simulink model "celp_ex_lsf"  (Simulink 6.1)
settings: Solver=FixedStepDiscrete  SolverMode=SingleTasking  StartTime=0.0  StopTime=300  RelTol=1e-3
PreLoadFcn:
  | load lpcvocoder.mat;
undefined symbols (not defined in the file): jet, magnitude, poly2lsf
libraries: simulink x16, dspcelplib x12, dspindex x9, dspstat3 x8, dspbuff3 x8, dspquant2 x6, dspmtrx3 x6, dsparch4 x4, dspsigops x4, dspmathops x4, dsplp x3, dspspect3 x3
(part 1 of 2)
settings Model: RequirementInfo=9  CovMetricSettings=d  Creator=The MathWorks Inc.  LastModifiedBy=igor  ExtModeTrigMode=oneshot  ExtModeArmWhenConnect=off  ExtModeAutoUpdateStatusClock=off  ProdHWDeviceType=Specified
settings DataIOCC: LimitDataPoints=off  SaveFormat=Structure  SaveOutput=off  SaveTime=off  SignalLoggingName=sigsOut
settings OptimizationCC: BlockReduction=off  BooleanDataType=off  InlineInvariantSignals=off
settings DebuggingCC: CheckExecutionContextPreStartOutputMsg=on  CheckExecutionContextRuntimeOutputMsg=on  InheritedTsInSrcMsg=none  IntegerOverflowMsg=none
settings HardwareCC: ProdHWDeviceType=Specified

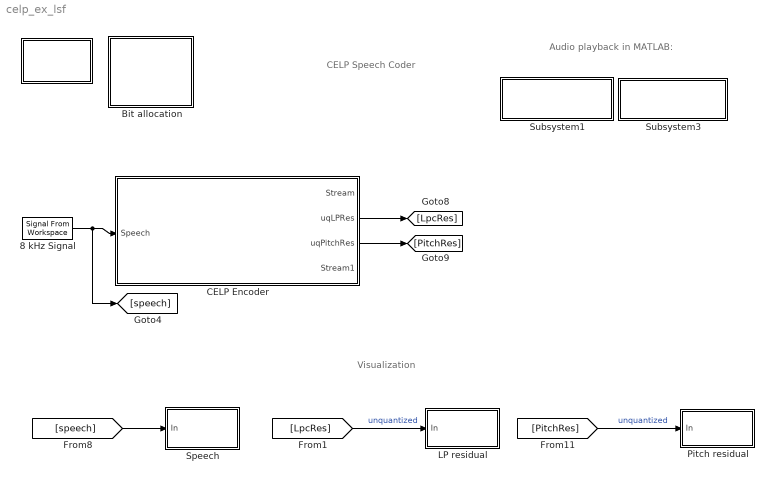
== system celp_ex_lsf ==
  note: CELP Speech Coder
  note: Visualization
  note: Audio playback in MATLAB:
  " " : Subsystem
      mask Type: CELP Coder Demo Info
      mask Display: disp('Info')
  "  Bit allocation" : Subsystem  mask(Bit Allocation){bitLSF1to3=10, bitLSF4to6=10, bitLSF7to10=10, bitD=7, bitBeta=6, bitSignGain=4, bitPhase=17, bitAlpha=6}
      mask prompts: bitLSF1to3 "Number of bits for 1st LSF subvector (1 to 3) (per frame):"; bitLSF4to6 "Number of bits for 2nd LSF subvector (4 to 6) (per frame):"; bitLSF7to10 "Number of bits for 3rd LSF subvector (7 to 10) (per frame):"; bitD "Number of bits for Pitch Delay, D (per subframe):"; bitBeta "Number of bits for Pitch Gain, Beta (per subframe):"; bitSignGain "Number of bits for sign of 4 FCB pulses (per subframe):"; bitPhase "Number of bits for position of 4 FCB pulses (per subframe):"; bitAlpha "Number of bits for FCB Gain, Alpha (per subframe):"
      mask help: Bit allocation for the speech coder designed for narrowband speech (sampling frequency 8 KHz) having a frame length of 160 samples and a subframe length of 40 samples (4 subframes per frame).
      mask StyleString: popup(10),popup(10),popup(10),popup(7),popup(6),popup(4),popup(17),popup(6)
      mask Display: disp('Bitrate\n9500 bps')
  8 kHz Signal : dspsrcs4/Signal From Workspace  X=speech2  Ts=1/8000  nsamps=160  OutputAfterFinalValue=Setting to zero
  CELP Encoder : Subsystem
      mask Display:
      | disp('CELP\nEncoder')
      | port_label('input',1,'Speech')
      | port_label('output',1,'Data Stream')
      | port_label('output',2,'LPC Residual')
      | port_label('output',3,'Pitch Residual')
      | port_label('output',4,'LSF')
  LP residual : Subsystem
      mask Display: disp('Spectrogram');
  Pitch residual : Subsystem
      mask Display: disp('Spectrogram');
  Speech : Subsystem
      mask Display: disp('Spectrogram');
  Subsystem1 : Subsystem
      settings: OpenFcn=if exist('Speech','var'), soundsc(Speech,8000); else errordlg('Data not found in workspace - reload demo model.','Signal Processing Blockset Demo Error'); end
      mask Display: disp('Original\nSignal')
  Subsystem3 : Subsystem
      settings: OpenFcn=if exist('y_lpc','var'), soundsc(y_lpc,8000); else uiwait(errordlg('You must run the simulation first.','Signal Processing Blockset Demo Error','modal')); end
      mask Display: disp('Processed\nSignal')
  wires:
  8 kHz Signal/1 -> CELP Encoder/1(Speech), [speech]
  CELP Encoder/2(uqLPRes) -> [LpcRes]
  CELP Encoder/3(uqPitchRes) -> [PitchRes]
  [speech] -> Speech/1(In)
  [LpcRes] -> LP residual/1(In)  "unquantized"
  [PitchRes] -> Pitch residual/1(In)  "unquantized"

== system celp_ex_lsf/  ==
  note: Code Excited Linear Prediction (CELP) speech coder demo
      |
      | This demo contains a CELP coder composed of an encoder and a decoder.
      |
      | In the encoder, we estimate the parameters of the short-term synthesis
      | filter, the long-term pitch filter and the innovation signal.
      |
      | Using the linear prediction (LP) analysis followed by the quantization and
      | the interpolation of the LSF parameters we calculate the synthesis filter
      | coefficients for each subframe.
      |
      | By applying open loop pitch analysis on the LPC residual signal in each
      | subframe we estimate the pitch predictor delay and the pitch gain
      | parameters.
      |
      | By applying a search on the pitch predictor residual we specify the
      | location and the signs of the FCB (Fixed Code Book) pulses and the FCB
      | gain.
      |
      | To illustrate how the LPC and the pitch analyses remove the short-term and
      | long-term redundancies in the speech signal, the LPC and the pitch residual
      | signals are visualized.
      |
      | The decoder re-synthesizes the speech signal based on the CELP coder
      | parameters contained in the data stream.
      |
      | In this simulation, the speech signal is divided into frames of size 20 ms
      | (160 samples) and each frame is subdivided into four subframes of 5 ms (40
      | samples) each. The bit allocation for each parameter of the coder can be
      | found by double clicking on the 'Bit Allocation' block.
      |
      | The speech phrase used in this demo is from the Harvard list of
      | phonetically balanced sentences, list 14, phrase 8:
      | "Clothes and lodging are free to new men."

== system celp_ex_lsf/  Bit allocation ==

== system celp_ex_lsf/CELP Encoder ==
  Speech : Inport  Port=1  LatchInput=off
  DC bias removal : dsparch4/Digital Filter  DialogController=dspDDGCreate  DialogControllerArgs=DataTag0  TypePopup=IIR (poles & zeros)  IIRFiltStruct=Direct form II transposed  AllPoleFiltStruct=Direct form  FIRFiltStruct=Direct form  CoeffSource=Specify via dialog  NumCoeffs="[ 0.9201   -1.8401    0.9201]"  DenCoeffs="[ 1.0000   -1.8337    0.8465]"  BiQuadCoeffs=[1 0.3 0.4 1 0.1 0.2]  LatticeCoeffs=[0.2 0.4]  denIgnore=on  FiltPerSampPopup=One filter per frame  IC=0  ICnum=0  ICden=0  roundingMode=Floor  overflowMode=off  ScaleValues=1  scaleValueFracLength=14  stageInFracLength=15  stageOutFracLength=15
  Data-Stream generation : simulink/Math Operations/Matrix Concatenation  numInports=6  catMethod=Horizontal
  Frame Analysis : Subsystem
  Reshape : simulink/Math Operations/Reshape  OutputDimensionality=Customize  OutputDimensions=[160,1]
  Subframe Analysis : Subsystem  TreatAsAtomicUnit=on
  Subframe to frame : simulink/Math Operations/Reshape  OutputDimensionality=Customize  OutputDimensions=[160,1]
  Stream : Outport
  uqLPRes : Outport  Port=2
  uqPitchRes : Outport  Port=3
  Stream1 : Outport  Port=4
  wires:
  Frame Analysis/2(LSF) -> Subframe Analysis/1(LSF)
  Subframe Analysis/1(Idx_D) -> Data-Stream generation/2
  DC bias removal/1 -> Frame Analysis/1(FilteredSp), Subframe Analysis/2(Speech)
  Subframe Analysis/6(uqLPRes) -> Reshape/1
  Subframe Analysis/7(uqPitchRes) -> Subframe to frame/1
  Frame Analysis/1(IdxLSF) -> Data-Stream generation/1, Stream1/1
  Subframe Analysis/2(Idx_Beta) -> Data-Stream generation/3
  Subframe Analysis/3(4Position) -> Data-Stream generation/4
  Subframe Analysis/4(4SignBit) -> Data-Stream generation/5
  Subframe Analysis/5(Idx_FCBgain) -> Data-Stream generation/6
  Data-Stream generation/1 -> Stream/1
  Speech/1 -> DC bias removal/1
  Reshape/1 -> uqLPRes/1
  Subframe to frame/1 -> uqPitchRes/1

== system celp_ex_lsf/LP residual ==
  In : Inport  Port=1  LatchInput=off
  Buffer1 : dspbuff3/Buffer  N=256  V=256-160  ic=0
  Buffer3 : dspbuff3/Buffer  N=96  V=94  ic=-70
  Selector1 : Selector  Elements=1:128  InputPortWidth=256
  Short-Time FFT1 : dspspect3/Periodogram  wintype=Hamming  Rs=50  beta=5  winsamp=Periodic  inheritFFT=on  fftsize=256  navg=2
  Spectrogram : dspsnks4/Matrix Viewer  ImageParams=off  CMapStr=jet(256)  AxisColorbar=on  AxisParams=off  AxisOrigin=Lower left corner  XLabel=Time Index  YLabel=Frequency Index  ZLabel=dB Magnitude  FigPos=[438 210 380 320]  AxisZoom=off
      settings: YMin=-70  YMax=15
  Transpose1 : dspmtrx3/Transpose  Hermitian=off  overflowFlag=on
  dB Conversion1 : dspmathops/dB Conversion  dBtype=dB  intype=Amplitude  R=1  fuzz=on
  wires:
  In/1 -> Buffer1/1
  Transpose1/1 -> Spectrogram/1
  Buffer3/1 -> Transpose1/1
  dB Conversion1/1 -> Buffer3/1
  Short-Time FFT1/1 -> Selector1/1
  Selector1/1 -> dB Conversion1/1
  Buffer1/1 -> Short-Time FFT1/1

== system celp_ex_lsf/Pitch residual ==
  In : Inport  Port=1  LatchInput=off
  Buffer1 : dspbuff3/Buffer  N=256  V=256-160  ic=0
  Buffer3 : dspbuff3/Buffer  N=96  V=94  ic=-70
  Selector1 : Selector  Elements=1:128  InputPortWidth=256
  Short-Time FFT1 : dspspect3/Periodogram  wintype=Hamming  Rs=50  beta=5  winsamp=Periodic  inheritFFT=on  fftsize=128  navg=2
  Spectrogram : dspsnks4/Matrix Viewer  ImageParams=off  CMapStr=jet(256)  AxisColorbar=on  AxisParams=on  AxisOrigin=Lower left corner  XLabel=Time Index  YLabel=Frequency Index  ZLabel=dB Magnitude  FigPos=[826 210 380 320]  AxisZoom=off
      settings: YMin=-70  YMax=15
  Transpose1 : dspmtrx3/Transpose  Hermitian=off  overflowFlag=on
  dB Conversion1 : dspmathops/dB Conversion  dBtype=dB  intype=Amplitude  R=1  fuzz=on
  wires:
  Buffer1/1 -> Short-Time FFT1/1
  Selector1/1 -> dB Conversion1/1
  Short-Time FFT1/1 -> Selector1/1
  dB Conversion1/1 -> Buffer3/1
  Buffer3/1 -> Transpose1/1
  Transpose1/1 -> Spectrogram/1
  In/1 -> Buffer1/1

== system celp_ex_lsf/Speech ==
  In : Inport  Port=1  LatchInput=off
  Buffer1 : dspbuff3/Buffer  N=256  V=256-160  ic=0
  Buffer3 : dspbuff3/Buffer  N=96  V=94  ic=-70
  Selector1 : Selector  Elements=1:128  InputPortWidth=256
  Short-Time FFT1 : dspspect3/Periodogram  wintype=Hamming  Rs=50  beta=5  winsamp=Periodic  inheritFFT=on  fftsize=256  navg=2
  Spectrogram : dspsnks4/Matrix Viewer  ImageParams=off  CMapStr=jet(256)  AxisColorbar=on  AxisParams=off  AxisOrigin=Lower left corner  XLabel=Time Index  YLabel=Frequency Index  ZLabel=dB Magnitude  FigPos=[50 210 380 320]  AxisZoom=off
      settings: YMin=-70  YMax=15
  Transpose1 : dspmtrx3/Transpose  Hermitian=off  overflowFlag=on
  dB Conversion1 : dspmathops/dB Conversion  dBtype=dB  intype=Amplitude  R=1  fuzz=on
  wires:
  Buffer1/1 -> Short-Time FFT1/1
  Selector1/1 -> dB Conversion1/1
  Short-Time FFT1/1 -> Selector1/1
  dB Conversion1/1 -> Buffer3/1
  Buffer3/1 -> Transpose1/1
  Transpose1/1 -> Spectrogram/1
  In/1 -> Buffer1/1

== system celp_ex_lsf/Subsystem1 ==

== system celp_ex_lsf/Subsystem3 ==

== system celp_ex_lsf/CELP Encoder/Frame Analysis ==
  FilteredSp : Inport  Port=1  LatchInput=off
  " " : Subsystem
      mask Type: CELP Coder Demo Info
      mask Display: disp('Info')
  Classical LPC analysis : Subsystem
      mask Display:
      | disp('LPC\nAnalysis');
      | port_label('input',1,'speech');
      | port_label('output',1,'LPC');
  LSF Interpolation : Subsystem
  LSF Vector Quantization : Subsystem
  IdxLSF : Outport
  LSF : Outport  Port=2
  wires:
  Classical LPC analysis/1(LPC) -> LSF Vector Quantization/1(LPC)
  LSF Vector Quantization/1(qLSF) -> LSF Interpolation/1(LSF)
  FilteredSp/1 -> Classical LPC analysis/1(Speech)
  LSF Interpolation/1(LSFinterp) -> LSF/1
  LSF Vector Quantization/2(IdxLSF) -> IdxLSF/1

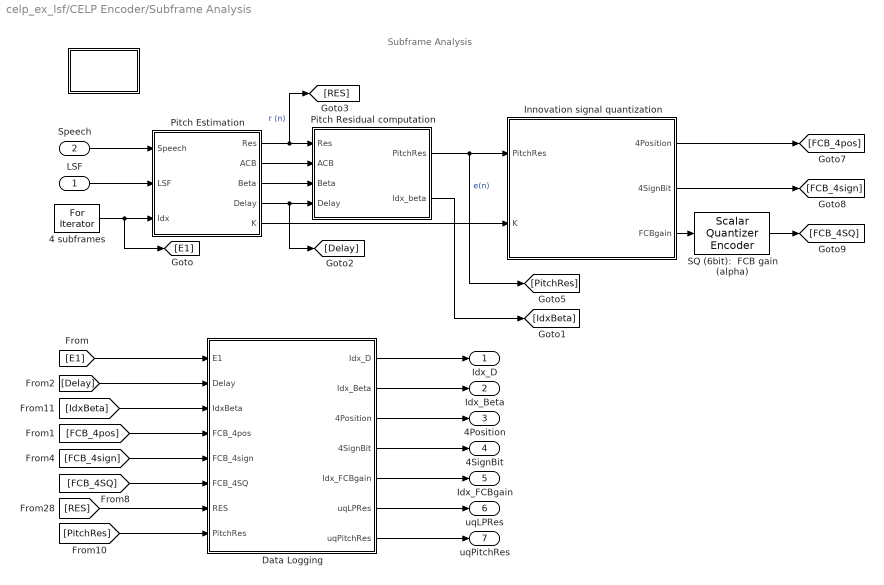
== system celp_ex_lsf/CELP Encoder/Subframe Analysis ==
  note: Subframe Analysis
  LSF : Inport  Port=1  LatchInput=off
  Speech : Inport  Port=2  LatchInput=off
  " " : Subsystem
      mask Type: CELP Coder Demo Info
      mask Display: disp('Info')
  4 subframes : ForIterator  IterationLimit=4
  Data Logging : Subsystem
  Innovation signal quantization : Subsystem
      mask Display:
      | disp('Pitch\nResidual\nQuantizer');
      | port_label('input',1,'PitchRes');
      | port_label('input',2,'K');
      | port_label('output',1,'4Position');
      | port_label('output',2,'4SignBit');
      | port_label('output',3,'FCBgain');
  Pitch Estimation : Subsystem
  Pitch Residual computation : Subsystem
  SQ (6bit):  FCB gain (alpha) : dspquant2/Scalar Quantizer Encoder  paramSrc=Specify via dialog  partType=Unbounded  BBoundary=[1:10]  UBoundary="[-0.050059   -0.040204   -0.034578   -0.030251   -0.025995   -0.022746   -0.018697    -0.01444   -0.011291  -0.0087536  -0.0064746  -0.0044205  -0.0026578  -0.0012629 -0.00019423  0.00069587   0.0015648   0.0025058   0.0035148   0.0045985   0.0057637   0.0070046   0.0083263   0.0097388    0.011246    0.012893    0.014707    0.016689    0.018853    0.021216    0.023812    0.026607    0.029663    0.032998    0.036494    0.040261    0.044496    0.049179    0.054286    0.059915    0.066008    0.072462    0.079015    0.085986    0.092922    0.098403     0.10238     0.10603     0.10996     0.11383      0.1172     0.12041     0.12439     0.12834     0.13191     0.13575     0.14011     0.14347     0.14644     0.15537     0.16404     0.16779     0.17495]"  SearchMethod=Binary  tieBreakRule=Choose the lower index  outQU=off  outQError=off  codebook="[-1082.3569     -246.64044     -206.60177     -119.68735     -118.12987     -109.71395     -107.74187     -101.39102     -96.836918     -91.269156     -86.372177     -83.198634     -82.501047     -77.265358     -76.499561     -74.506154     -73.162943     -72.064354     -69.588398     -67.441995     -64.571558     -63.949501     -62.716478     -61.876738     -61.311021     -60.518343     -58.650854     -57.975792     -56.936942     -56.282238     -55.386427     -54.862852     -53.494072      -52.94422     -52.032961      -50.72662     -48.968103      -46.10807       -42.6265     -39.065568     -34.843913     -30.198965     -25.969732     -21.578415     -17.256677     -13.047571     -8.5748944     -4.8378646     -2.2872972    -0.86065481    -0.37978458     0.45579633     0.94262874      4.3421606      12.379451      23.629803       37.40066      54.817595      74.624825      93.641473      110.49643      136.97269      179.36351      233.98073]"  outStatus=off  invalidin=Clip  idtype=int32  roundingMode=Floor  overflowMode=off
  Idx_D : Outport
  Idx_Beta : Outport  Port=2
  4Position : Outport  Port=3
  4SignBit : Outport  Port=4
  Idx_FCBgain : Outport  Port=5
  uqLPRes : Outport  Port=6
  uqPitchRes : Outport  Port=7
  wires:
  4 subframes/1 -> [E1], Pitch Estimation/3(Idx)
  Speech/1 -> Pitch Estimation/1(Speech)
  LSF/1 -> Pitch Estimation/2(LSF)
  Data Logging/1(Idx_D) -> Idx_D/1
  [Delay] -> Data Logging/2(Delay)
  Pitch Residual computation/1(PitchRes) -> [PitchRes], Innovation signal quantization/1(PitchRes)  "e(n)"
  Data Logging/2(Idx_Beta) -> Idx_Beta/1
  Data Logging/6(uqLPRes) -> uqLPRes/1
  Data Logging/7(uqPitchRes) -> uqPitchRes/1
  [PitchRes] -> Data Logging/8(PitchRes)
  [RES] -> Data Logging/7(RES)
  Pitch Estimation/5(K) -> Innovation signal quantization/2(K)
  Innovation signal quantization/3(FCBgain) -> SQ (6bit):  FCB gain (alpha)/1
  Data Logging/5(Idx_FCBgain) -> Idx_FCBgain/1
  Data Logging/3(4Position) -> 4Position/1
  Data Logging/4(4SignBit) -> 4SignBit/1
  Pitch Estimation/1(Res) -> Pitch Residual computation/1(Res), [RES]  "r (n)"
  Pitch Estimation/2(ACB) -> Pitch Residual computation/2(ACB)
  Pitch Estimation/3(Beta) -> Pitch Residual computation/3(Beta)
  Pitch Estimation/4(Delay) -> Pitch Residual computation/4(Delay), [Delay]
  Innovation signal quantization/1(4Position) -> [FCB_4pos]
  [FCB_4pos] -> Data Logging/4(FCB_4pos)
  Innovation signal quantization/2(4SignBit) -> [FCB_4sign]
  [FCB_4sign] -> Data Logging/5(FCB_4sign)
  SQ (6bit):  FCB gain (alpha)/1 -> [FCB_4SQ]
  [FCB_4SQ] -> Data Logging/6(FCB_4SQ)
  Pitch Residual computation/2(Idx_beta) -> [IdxBeta]
  [IdxBeta] -> Data Logging/3(IdxBeta)
  [E1] -> Data Logging/1(E1)

== system celp_ex_lsf/CELP Encoder/Frame Analysis/  ==
  note: Frame analysis is composed of three steps:
      |
      | 1. Classical LPC analysis
      | 2. Split vector quantization of LSF vector
      | 3. LSF interpolation

== system celp_ex_lsf/CELP Encoder/Frame Analysis/Classical LPC analysis ==
  note: LPC Analysis
  Speech : Inport  Port=1  LatchInput=off
  " " : Subsystem
      mask Type: CELP Coder Demo Info
      mask Display: disp('Info')
  Autocorrelation : dspstat3/Autocorrelation  DialogController=dspDDGCreate  DialogControllerArgs=DataTag1  AllPositiveLags=off  maxlag=10  bias=Biased  domain=Time  roundingMode=Floor  overflowMode=off
  Bandwidth Expansion : Subsystem  mask(Bandwidth Expansion){alpha=0.994}
      mask prompts: alpha "Bandwidth expansion factor:"
      mask help:
      | Generate autoregressive (AR) polynomial with bandwidth expanded relative to the bandwidth of the input AR polynomial.
      |
      | By reducing the radius of the roots in an autoregressive polynomial (i.e., scaling them towards the origin of the Z-plane), the bandwidth of the spectral peaks in the frequency response is expanded (flattened).  This operation is often referred to as "bandwidth expansion".
      |
      | Bandwidth expansion factor must be in the range [0,1], where 1.0 yields no changes to the roots of the polynomial.
      mask Help: web(dspbhelp);
      mask Display: fprintf('Bandwidth\nExpansion\n%g', alpha)
  Levinson- Durbin : dspsolvers/Levinson-Durbin  DialogController=dspDDGCreate  DialogControllerArgs=DataTag3  coeffOutFcn=A  outP=off  zeroInpHandling=on  firstCoeffMode=Binary point scaling  firstCoeffWordLength=16  firstCoeffFracLength=15  secondCoeffMode=Binary point scaling  secondCoeffWordLength=16  secondCoeffFracLength=15  roundingMode=Floor  overflowMode=off
      settings: allowOverrides=off
  Overlap Analysis Windows : dspbuff3/Buffer  N=240  V=80  ic=0
  Window : dspsigops/Window Function  DialogController=dspDDGCreate  DialogControllerArgs=DataTag4  winmode=Apply window to input  wintype=Hamming  sampmode=Continuous  samptime=1  N=64  Rs=50  beta=10  winsamp=Symmetric  UserWindow=hamming  OptParams=off  UserParams={1.0}  dataType=double  isSigned=on  wordLen=16  udDataType=sfix(16)  fracBitsMode=Best precision  numFracBits=15  roundingMode=Floor  overflowMode=off
  LPC : Outport
  wires:
  Overlap Analysis Windows/1 -> Window/1
  Autocorrelation/1 -> Levinson- Durbin/1
  Window/1 -> Autocorrelation/1
  Speech/1 -> Overlap Analysis Windows/1
  Levinson- Durbin/1 -> Bandwidth Expansion/1(In1)
  Bandwidth Expansion/1(Out1) -> LPC/1

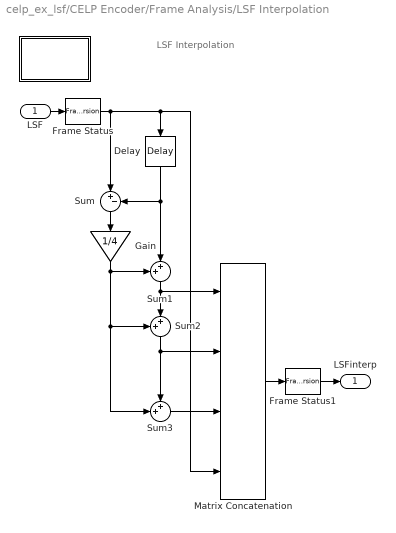
== system celp_ex_lsf/CELP Encoder/Frame Analysis/LSF Interpolation ==
  note: LSF Interpolation
  LSF : Inport  Port=1  LatchInput=off
  " " : Subsystem
      mask Type: CELP Coder Demo Info
      mask Display: disp('Info')
  Delay : dspsigops/Delay  Orientation=down  dly_unit=Frames  delay=1  ic_detail=on  dif_ic_for_ch=off  dif_ic_for_dly=on  ic=(poly2lsf([1 zeros(1,10)])).'  reset_popup=None
  Frame Status : FrameConversion
  Frame Status1 : FrameConversion  OutFrame=Sample based
  Gain : Gain  Orientation=down  Gain=1/4  SaturateOnIntegerOverflow=on
  Matrix Concatenation : simulink/Math Operations/Matrix Concatenation  numInports=4  catMethod=Horizontal
  Sum : Sum  Orientation=down  Inputs=|+-  SaturateOnIntegerOverflow=on
  Sum1 : Sum  Orientation=down  Inputs=++|  SaturateOnIntegerOverflow=on
  Sum2 : Sum  Orientation=down  Inputs=++|  SaturateOnIntegerOverflow=on
  Sum3 : Sum  Inputs=++|  SaturateOnIntegerOverflow=on
  LSFinterp : Outport
  wires:
  Frame Status/1 -> Sum/1, Delay/1, Matrix Concatenation/4
  Sum/1 -> Gain/1
  Sum1/1 -> Matrix Concatenation/1, Sum2/2
  Matrix Concatenation/1 -> Frame Status1/1
  Sum2/1 -> Sum3/1, Matrix Concatenation/2
  Sum3/1 -> Matrix Concatenation/3
  Delay/1 -> Sum1/2, Sum/2
  Gain/1 -> Sum1/1, Sum2/1, Sum3/2
  LSF/1 -> Frame Status/1
  Frame Status1/1 -> LSFinterp/1

== system celp_ex_lsf/CELP Encoder/Frame Analysis/LSF Vector Quantization ==
  note: Split Vector Quantization of LSF vector
  LPC : Inport  Port=1  LatchInput=off
  " " : Subsystem
      mask Type: CELP Coder Demo Info
      mask Display: disp('Info')
  LPC to LSF  conversion : dsplp/LPC to LSF//LSP Conversion  output=LSF in range (0 pi)  NSteps=64  NBisects=4  RootStatus=off  correction=off  lastLSP=off  error=Ignore
  LSF Split VQ. : Subsystem
  Paliwal Weight  Computation : Subsystem
  Reshape1 : simulink/Math Operations/Reshape  OutputDimensionality=Column vector  OutputDimensions=[1,1]
  qLSF : Outport
  IdxLSF : Outport  Port=2
  wires:
  LPC/1 -> Reshape1/1
  Paliwal Weight  Computation/1(Weights) -> LSF Split VQ./2(W1to10)
  Reshape1/1 -> LPC to LSF  conversion/1, Paliwal Weight  Computation/2(LPC)
  LPC to LSF  conversion/1 -> Paliwal Weight  Computation/1(LSF), LSF Split VQ./1(U1to10)
  LSF Split VQ./1(qLSF) -> qLSF/1
  LSF Split VQ./2(IdxLSF) -> IdxLSF/1

== system celp_ex_lsf/CELP Encoder/Subframe Analysis/  ==
  note: Subframe analysis is composed of three steps:
      |
      | 1. Pitch estimation
      | 2. Pitch residual (innovation signal) computation
      | 3. Innovation signal quantization using fixed codebook

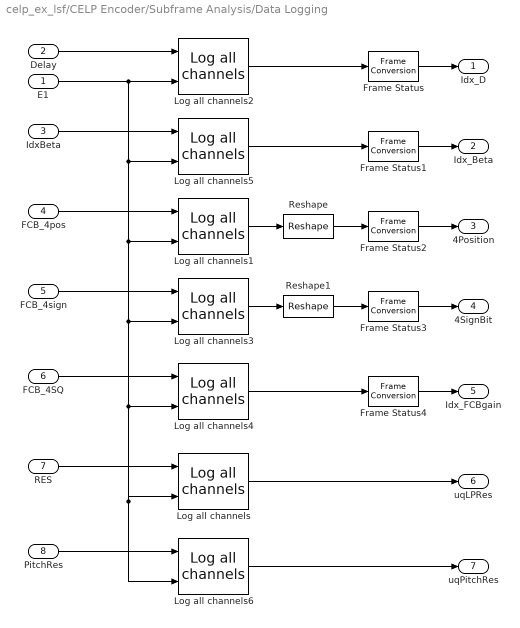
== system celp_ex_lsf/CELP Encoder/Subframe Analysis/Data Logging ==
  E1 : Inport  Port=1  LatchInput=off
  Delay : Inport  Port=2  LatchInput=off
  IdxBeta : Inport  Port=3  LatchInput=off
  FCB_4pos : Inport  Port=4  LatchInput=off
  FCB_4sign : Inport  Port=5  LatchInput=off
  FCB_4SQ : Inport  Port=6  LatchInput=off
  RES : Inport  Port=7  LatchInput=off
  PitchRes : Inport  Port=8  LatchInput=off
  Frame Status{,1..4} (5 alike) : FrameConversion  OutFrame=Sample based
  Log all channels : dspcelplib/Log all channels  outType=Matrix  numRow=40  numCol=4  dType=double
  Log all channels1 : dspcelplib/Log all channels  outType=Matrix  numRow=4  numCol=4  dType=int32
  Log all channels2 : dspcelplib/Log all channels  outType=Row vector  numRow=40  numCol=4  dType=int32
  Log all channels3 : dspcelplib/Log all channels  outType=Matrix  numRow=4  numCol=4  dType=int32
  Log all channels4 : dspcelplib/Log all channels  outType=Row vector  numRow=40  numCol=4  dType=int32
  Log all channels5 : dspcelplib/Log all channels  outType=Row vector  numRow=40  numCol=4  dType=int32
  Log all channels6 : dspcelplib/Log all channels  outType=Matrix  numRow=40  numCol=4  dType=double
  Reshape : simulink/Math Operations/Reshape  OutputDimensionality=Customize  OutputDimensions=[1,16]
  Reshape1 : simulink/Math Operations/Reshape  OutputDimensionality=Customize  OutputDimensions=[1,16]
  Idx_D : Outport
  Idx_Beta : Outport  Port=2
  4Position : Outport  Port=3
  4SignBit : Outport  Port=4
  Idx_FCBgain : Outport  Port=5
  uqLPRes : Outport  Port=6
  uqPitchRes : Outport  Port=7
  wires:
  E1/1 -> Log all channels/2, Log all channels6/2, Log all channels4/2, Log all channels3/2, Log all channels1/2, Log all channels5/2, Log all channels2/2
  Log all channels1/1 -> Reshape/1
  Log all channels3/1 -> Reshape1/1
  Delay/1 -> Log all channels2/1
  Log all channels2/1 -> Frame Status/1
  IdxBeta/1 -> Log all channels5/1
  Log all channels5/1 -> Frame Status1/1
  FCB_4pos/1 -> Log all channels1/1
  Reshape/1 -> Frame Status2/1
  FCB_4sign/1 -> Log all channels3/1
  Reshape1/1 -> Frame Status3/1
  FCB_4SQ/1 -> Log all channels4/1
  Log all channels4/1 -> Frame Status4/1
  RES/1 -> Log all channels/1
  Log all channels/1 -> uqLPRes/1
  PitchRes/1 -> Log all channels6/1
  Log all channels6/1 -> uqPitchRes/1
  Frame Status/1 -> Idx_D/1
  Frame Status1/1 -> Idx_Beta/1
  Frame Status2/1 -> 4Position/1
  Frame Status3/1 -> 4SignBit/1
  Frame Status4/1 -> Idx_FCBgain/1

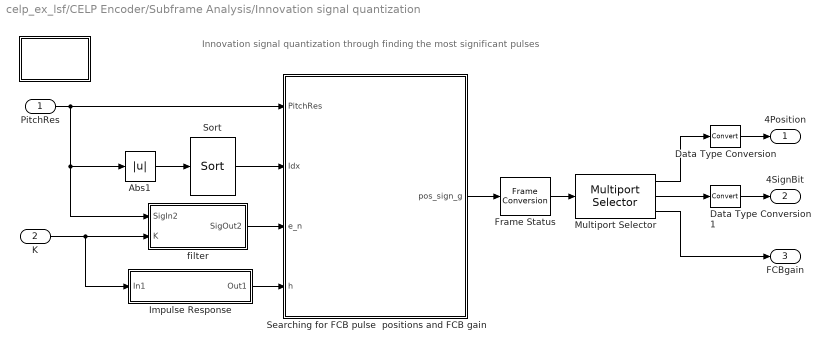
== system celp_ex_lsf/CELP Encoder/Subframe Analysis/Innovation signal quantization ==
  note: Innovation signal quantization through finding the most significant pulses
  PitchRes : Inport  Port=1  LatchInput=off
  K : Inport  Port=2  LatchInput=off
  " " : Subsystem
      mask Type: CELP Coder Demo Info
      mask Display: disp('Info')
  Abs1 : Abs  SaturateOnIntegerOverflow=on
  Data Type Conversion : DataTypeConversion  OutDataTypeMode=int32  SaturateOnIntegerOverflow=on  RndMeth=Zero
  Data Type Conversion1 : DataTypeConversion  OutDataTypeMode=int32  SaturateOnIntegerOverflow=on  RndMeth=Zero
  Frame Status : FrameConversion  OutFrame=Sample based
  Impulse Response : Subsystem
      mask Display:
      | disp('Impulse Response');
      | port_label('input',1,'K');
      | port_label('output',1,'h');
  Multiport Selector : dspindex/Multiport Selector  rowsOrCols=Rows  idxCellArray={ 1:4,5:8,9 }  idxErrMode=Generate Error
  Searching for FCB pulse  positions and FCB gain : Subsystem  TreatAsAtomicUnit=on
  Sort : dspstat3/Sort  DialogController=dspDDGCreate  DialogControllerArgs=DataTag9  otype=Index  dir=Descending  sortAlg=Quick sort  roundingMode=Floor  overflowMode=off
  filter : Subsystem  TreatAsAtomicUnit=on
      mask Display:
      | disp('Zero State\nIIR Lattice\nFilter');
      | port_label('input',1,'In');
      | port_label('input',2,'K');
      | port_label('output',1,'Out');
  4Position : Outport
  4SignBit : Outport  Port=2
  FCBgain : Outport  Port=3
  wires:
  Impulse Response/1(Out1) -> Searching for FCB pulse  positions and FCB gain/4(h)
  filter/1(SigOut2) -> Searching for FCB pulse  positions and FCB gain/3(e_n)
  K/1 -> Impulse Response/1(In1), filter/2(K)
  Multiport Selector/3 -> FCBgain/1
  Data Type Conversion1/1 -> 4SignBit/1
  Data Type Conversion/1 -> 4Position/1
  Sort/1 -> Searching for FCB pulse  positions and FCB gain/2(Idx)
  Abs1/1 -> Sort/1
  PitchRes/1 -> filter/1(SigIn2), Abs1/1, Searching for FCB pulse  positions and FCB gain/1(PitchRes)
  Multiport Selector/2 -> Data Type Conversion1/1
  Multiport Selector/1 -> Data Type Conversion/1
  Searching for FCB pulse  positions and FCB gain/1(pos_sign_g) -> Frame Status/1
  Frame Status/1 -> Multiport Selector/1

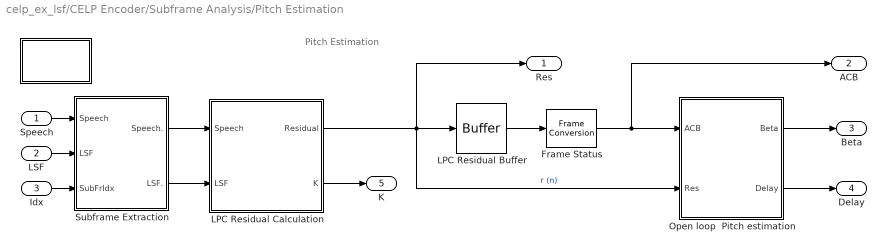
== system celp_ex_lsf/CELP Encoder/Subframe Analysis/Pitch Estimation ==
  note: Pitch Estimation
  Speech : Inport  Port=1  LatchInput=off
  LSF : Inport  Port=2  LatchInput=off
  Idx : Inport  Port=3  LatchInput=off
  " " : Subsystem
      mask Type: CELP Coder Demo Info
      mask Display: disp('Info')
  Frame Status : FrameConversion  OutFrame=Sample based
  LPC Residual Buffer : dspbuff3/Buffer  N=128+40+20-1  V=187-40  ic=0
  LPC Residual Calculation : Subsystem
  Open loop  Pitch estimation : Subsystem
  Subframe Extraction : Subsystem
  Res : Outport
  ACB : Outport  Port=2
  Beta : Outport  Port=3
  Delay : Outport  Port=4
  K : Outport  Port=5
  wires:
  Subframe Extraction/1(Speech.) -> LPC Residual Calculation/1(Speech)
  Subframe Extraction/2(LSF.) -> LPC Residual Calculation/2(LSF)
  LPC Residual Calculation/1(Residual) -> LPC Residual Buffer/1, Open loop  Pitch estimation/2(Res), Res/1  "r (n)"
  LPC Residual Buffer/1 -> Frame Status/1
  Speech/1 -> Subframe Extraction/1(Speech)
  Open loop  Pitch estimation/1(Beta) -> Beta/1
  LSF/1 -> Subframe Extraction/2(LSF)
  LPC Residual Calculation/2(K) -> K/1
  Idx/1 -> Subframe Extraction/3(SubFrIdx)
  Open loop  Pitch estimation/2(Delay) -> Delay/1
  Frame Status/1 -> ACB/1, Open loop  Pitch estimation/1(ACB)

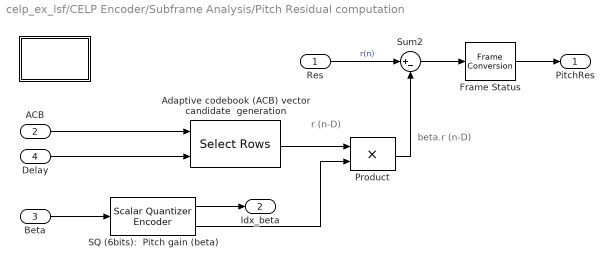
== system celp_ex_lsf/CELP Encoder/Subframe Analysis/Pitch Residual computation ==
  note: r (n-D)
  note: beta.r (n-D)
  Res : Inport  Port=1  LatchInput=off
  ACB : Inport  Port=2  LatchInput=off
  Beta : Inport  Port=3  LatchInput=off
  Delay : Inport  Port=4  LatchInput=off
  " " : Subsystem
      mask Type: CELP Coder Demo Info
      mask Display: disp('Info')
  Adaptive codebook (ACB) vector candidate  generation : dspcelplib/Select Rows  numRows=40
  Frame Status : FrameConversion  OutFrame=Sample based
  Product : Product  SaturateOnIntegerOverflow=on  InputSameDT=on
  SQ (6bits):  Pitch gain (beta) : dspquant2/Scalar Quantizer Encoder  paramSrc=Specify via dialog  partType=Unbounded  BBoundary=[1:10]  UBoundary="[-664.4987     -226.6211     -163.1446     -118.9086     -113.9219     -108.7279     -104.5664     -99.11397     -94.05304     -88.82067     -84.78541     -82.84984      -79.8832     -76.88246     -75.50286     -73.83455     -72.61365     -70.82638      -68.5152     -66.00678     -64.26053     -63.33299     -62.29661     -61.59388     -60.91468      -59.5846     -58.31332     -57.45637     -56.60959     -55.83433     -55.12464     -54.17846     -53.21915     -52.48859     -51.37979     -49.84736     -47.53809     -44.36728     -40.84603     -36.95474     -32.52144     -28.08435     -23.77407     -19.41755     -15.15212     -10.81123      -6.70638     -3.562581     -1.573976    -0.6202197    0.03800587     0.6992125      2.642395      8.360806      18.00463      30.51523      46.10913      64.72121      84.13315       102.069      123.7346      158.1681      206.6721]"  SearchMethod=Binary  tieBreakRule=Choose the lower index  outQU=on  outQError=off  codebook="[-1082.3569     -246.64044     -206.60177     -119.68735     -118.12987     -109.71395     -107.74187     -101.39102     -96.836918     -91.269156     -86.372177     -83.198634     -82.501047     -77.265358     -76.499561     -74.506154     -73.162943     -72.064354     -69.588398     -67.441995     -64.571558     -63.949501     -62.716478     -61.876738     -61.311021     -60.518343     -58.650854     -57.975792     -56.936942     -56.282238     -55.386427     -54.862852     -53.494072      -52.94422     -52.032961      -50.72662     -48.968103      -46.10807       -42.6265     -39.065568     -34.843913     -30.198965     -25.969732     -21.578415     -17.256677     -13.047571     -8.5748944     -4.8378646     -2.2872972    -0.86065481    -0.37978458     0.45579633     0.94262874      4.3421606      12.379451      23.629803       37.40066      54.817595      74.624825      93.641473      110.49643      136.97269      179.36351      233.98073]"  outStatus=off  invalidin=Clip  idtype=int32  roundingMode=Floor  overflowMode=off
  Sum2 : Sum  Inputs=|+-  SaturateOnIntegerOverflow=on
  PitchRes : Outport
  Idx_beta : Outport  Port=2
  wires:
  ACB/1 -> Adaptive codebook (ACB) vector candidate  generation/1
  Sum2/1 -> Frame Status/1
  Res/1 -> Sum2/1  "r(n)"
  Delay/1 -> Adaptive codebook (ACB) vector candidate  generation/2
  Product/1 -> Sum2/2
  Adaptive codebook (ACB) vector candidate  generation/1 -> Product/1
  Beta/1 -> SQ (6bits):  Pitch gain (beta)/1
  SQ (6bits):  Pitch gain (beta)/2 -> Product/2
  SQ (6bits):  Pitch gain (beta)/1 -> Idx_beta/1
  Frame Status/1 -> PitchRes/1

== system celp_ex_lsf/CELP Encoder/Frame Analysis/Classical LPC analysis/  ==
  note: In this subsystem, LPC analysis is performed on a speech signal with a
      |
      | frame size of 30 ms (240 samples). This signal has an overlap of 10 ms
      |
      | (80 samples). Each frame is windowed using a Hamming window and 10th order
      |
      | autocorrelation coefficients are found. Using the Levinson Durbin
      |
      | algorithm, 10th order LP coefficients are calculated from the
      |
      | autocorrelation coefficients. Finally, the LP coefficients are modified
      |
      | using a bandwidth expansion block.

== system celp_ex_lsf/CELP Encoder/Frame Analysis/Classical LPC analysis/Bandwidth Expansion ==
  In1 : Inport  Port=1  LatchInput=off
  Window Function : dspsigops/Window Function  DialogController=dspDDGCreate  DialogControllerArgs=DataTag2  winmode=Apply window to input  wintype=User defined  sampmode=Continuous  samptime=1  N=64  Rs=50  beta=10  winsamp=Symmetric  UserWindow=bwexpwin  OptParams=on  UserParams=alpha  dataType=double  isSigned=on  wordLen=16  udDataType=sfix(16)  fracBitsMode=Best precision  numFracBits=15  roundingMode=Floor  overflowMode=off
  Out1 : Outport
  wires:
  In1/1 -> Window Function/1
  Window Function/1 -> Out1/1

== system celp_ex_lsf/CELP Encoder/Frame Analysis/LSF Interpolation/  ==
  note: In this subsystem the LSFs are interpolated, in order to:
      |
      | 1.  Avoid rapid changes in the LP parameters (LSFs) between successive frames
      |
      | 2.  Specify the synthesis filter parameters for each subframe.

== system celp_ex_lsf/CELP Encoder/Frame Analysis/LSF Vector Quantization/  ==
  note: In this portion of the subsystems, the following operations occur:
      |
      |
      | 1. Linear prediction (LP) coefficients are converted to line spectral
      |
      |    frequencies (LSFs). After quantization and interpolation, the stability
      |
      |    of the LP synthesis filter can be guaranteed in the LSF domain without
      |
      |    additional computation.
      |
      |
      | 2. Weighting factors used in the LSF quantization are calculated using the
      |
      |    method proposed by Paliwal and Atal*. In this method, the weight
      |
      |    assigned to a given LSF is proportional to the spectral sensitivity and
      |
      |    the value of the spectral envelope at the current LSF.
      |
      | *[ K.K. Paliwal and B.S. Atal, "Efficient vector quantization of LPC
      |
      |    parameters at 24 bits/frame," J. Acoust. Soc. Am., vol. 87, p. S39, 1990]

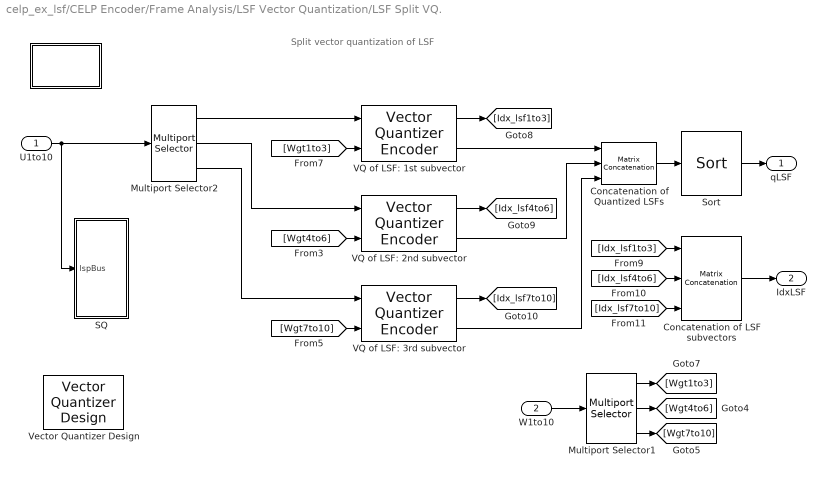
== system celp_ex_lsf/CELP Encoder/Frame Analysis/LSF Vector Quantization/LSF Split VQ. ==
  note: Split vector quantization of LSF
  U1to10 : Inport  Port=1  LatchInput=off
  W1to10 : Inport  Port=2  LatchInput=off
  " " : Subsystem
      mask Type: CELP Coder Demo Info
      mask Display: disp('Info')
  Concatenation of LSF subvectors : simulink/Math Operations/Matrix Concatenation  numInports=3  catMethod=Horizontal
  Concatenation of Quantized LSFs : simulink/Math Operations/Matrix Concatenation  numInports=3  catMethod=Vertical
  Multiport Selector1 : dspindex/Multiport Selector  rowsOrCols=Rows  idxCellArray={1:3,4:6,7:10}  idxErrMode=Clip Index
  Multiport Selector2 : dspindex/Multiport Selector  rowsOrCols=Rows  idxCellArray={1:3,4:6,7:10}  idxErrMode=Clip Index
  SQ : Subsystem
  Sort : dspstat3/Sort  DialogController=dspDDGCreate  DialogControllerArgs=DataTag5  otype=Value  dir=Ascending  sortAlg=Quick sort  roundingMode=Floor  overflowMode=off
  VQ of LSF: 1st subvector : dspquant2/Vector Quantizer Encoder  CBsource=Specify via dialog  codebook=CB_lsf1to3_10bit  distMeasure=Weighted squared error  wgtSrc=Input port  weights=[1 1 1]  tieBreakRule=Choose the lower index  outQU=on  outQError=off  idtype=int32  roundingMode=Floor  overflowMode=off
  VQ of LSF: 2nd subvector : dspquant2/Vector Quantizer Encoder  CBsource=Specify via dialog  codebook=CB_lsf4to6_10bit  distMeasure=Weighted squared error  wgtSrc=Input port  weights=[1 1 1]  tieBreakRule=Choose the lower index  outQU=on  outQError=off  idtype=int32  roundingMode=Floor  overflowMode=off
  VQ of LSF: 3rd subvector : dspquant2/Vector Quantizer Encoder  CBsource=Specify via dialog  codebook=CB_lsf7to10_10bit  distMeasure=Weighted squared error  wgtSrc=Input port  weights=[1 1 1]  tieBreakRule=Choose the lower index  outQU=on  outQError=off  idtype=int32  roundingMode=Floor  overflowMode=off
  Vector Quantizer Design : dspquant2/Vector Quantizer Design
  qLSF : Outport
  IdxLSF : Outport  Port=2
  wires:
  VQ of LSF: 1st subvector/2 -> Concatenation of Quantized LSFs/1
  VQ of LSF: 1st subvector/1 -> [Idx_lsf1to3]
  Multiport Selector2/2 -> VQ of LSF: 2nd subvector/1
  Multiport Selector2/3 -> VQ of LSF: 3rd subvector/1
  Multiport Selector1/2 -> [Wgt4to6]
  Multiport Selector1/3 -> [Wgt7to10]
  VQ of LSF: 2nd subvector/1 -> [Idx_lsf4to6]
  [Wgt7to10] -> VQ of LSF: 3rd subvector/2
  VQ of LSF: 3rd subvector/1 -> [Idx_lsf7to10]
  VQ of LSF: 2nd subvector/2 -> Concatenation of Quantized LSFs/2
  Concatenation of Quantized LSFs/1 -> Sort/1
  VQ of LSF: 3rd subvector/2 -> Concatenation of Quantized LSFs/3
  [Wgt4to6] -> VQ of LSF: 2nd subvector/2
  Multiport Selector1/1 -> [Wgt1to3]
  [Wgt1to3] -> VQ of LSF: 1st subvector/2
  [Idx_lsf1to3] -> Concatenation of LSF subvectors/1
  [Idx_lsf4to6] -> Concatenation of LSF subvectors/2
  [Idx_lsf7to10] -> Concatenation of LSF subvectors/3
  W1to10/1 -> Multiport Selector1/1
  U1to10/1 -> Multiport Selector2/1, SQ/1(lspBus)
  Sort/1 -> qLSF/1
  Concatenation of LSF subvectors/1 -> IdxLSF/1
  Multiport Selector2/1 -> VQ of LSF: 1st subvector/1

== system celp_ex_lsf/CELP Encoder/Frame Analysis/LSF Vector Quantization/Paliwal Weight  Computation ==
  note: Calculation of Perceptual Weighting Factors
  LSF : Inport  Port=1  LatchInput=off
  LPC : Inport  Port=2  LatchInput=off
  " " : Subsystem
      mask Type: CELP Coder Demo Info
      mask Display: disp('Info')
  Constant : Constant  Orientation=up  Value=0.15  VectorParams1D=off  SampleTime=-1
  Gain : Gain  Gain=-1
  Gain1 : Gain  Gain=[ones(1,8) 0.8 0.4]
  LPCpowSpec : Subsystem
  Math Function : Math  Operator=pow  SaturateOnIntegerOverflow=on
  Reshape : simulink/Math Operations/Reshape  OutputDimensionality=Column vector  OutputDimensions=[1,1]
  Submatrix : dspmtrx3/Submatrix  RowSpan=Range of rows  RowStartMode=Index  RowStartIndex=2  RowEndMode=Last  RowEndIndex=1  ColSpan=All columns  ColStartMode=First  ColStartIndex=1  ColEndMode=Last  ColEndIndex=1
  Weights : Outport
  wires:
  LPCpowSpec/1(Out) -> Math Function/1
  Constant/1 -> Math Function/2
  Math Function/1 -> Gain1/1
  Gain1/1 -> Reshape/1
  LSF/1 -> LPCpowSpec/2(LSF)
  Reshape/1 -> Weights/1
  Submatrix/1 -> Gain/1
  LPC/1 -> Submatrix/1
  Gain/1 -> LPCpowSpec/1(PC)

== system celp_ex_lsf/CELP Encoder/Subframe Analysis/Innovation signal quantization/  ==
  note: In this subsystem, the four "most significant pulses" are found from a
      |
      | subframe of length 40. Also, FCB gain is computed.
      |
      |
      |
      | 1. The absolute values of the 40 subframe samples are sorted in descending
      |
      | order. Their original positions are stored in a variable that has the
      |
      | following format: pos = [pos1, pos2, ..., pos40]. Here, pos1 stores the
      |
      | position of the largest valued sample, pos2 stores the position of the
      |
      | second largest valued sample, and so on.
      |
      |
      | 2.  The first four dominant samples are replaced by a +1 or a -1, where +1
      |
      | represents a positive sample and  -1 represents a negative sample. The
      |
      | other 36 samples are replaced by zeros. For example, a +1 or a -1 would be
      |
      | located at positions pos1, pos2, pos3, and pos4, and zeros would occupy the
      |
      | other positions.
      |
      |
      | 3. The zero-state response of the synthesis filter 1/A(z) to the original
      |
      | pitch residual signal is computed.
      |
      | 4. The zero-state response of the synthesis filter 1/A(z) to the quantized
      |
      | pitch residual signal is computed using the method of sparse filtering.
      |
      | Here, first the impulse response of the filter is calculated. Then the
      |
      | impulse response is convolved with the sparse representation of the
      |
      | quantized pitch residual signal.
      |
      |
      | 5. Steps 2 and 4 are repeated with four new samples from positions pos2,
      |
      | pos3, pos4, and pos5.
      |
      |
      |
      | This process is repeated for all 37 combinations of the positions. The set
      |
      | of four positions that minimize the error between the zero state response
      |
      | to the original pitch residual signal and the zero state response to the
      |
      | quantized pitch residual are the four "most significant pulses".

== system celp_ex_lsf/CELP Encoder/Subframe Analysis/Innovation signal quantization/Impulse Response ==
  In1 : Inport  Port=1  LatchInput=off
  DSP Constant : dspsrcs4/DSP Constant  Value=[1;zeros(39,1)]  SampleMode=Discrete  discreteOutput=Frame-based  continuousOutput=Sample-based  sampTime=1  framePeriod=-1  dataType=Inherit from 'Constant value'  isSigned=on  wordLen=16  udDataType=sfix(16)  fracBitsMode=Best precision  numFracBits=15  InterpretAs1D=-inf  Ts=-inf  FramebasedOutput=-inf
  For Iterator Subsystem2 : Subsystem  TreatAsAtomicUnit=on
      mask Display:
      | disp('Zero State\nIIR Lattice\nFilter');
      | port_label('input',1,'In');
      | port_label('input',2,'K');
      | port_label('output',1,'Out');
  Out1 : Outport
  wires:
  For Iterator Subsystem2/1(SigOut2) -> Out1/1
  In1/1 -> For Iterator Subsystem2/2(K)
  DSP Constant/1 -> For Iterator Subsystem2/1(SigIn2)

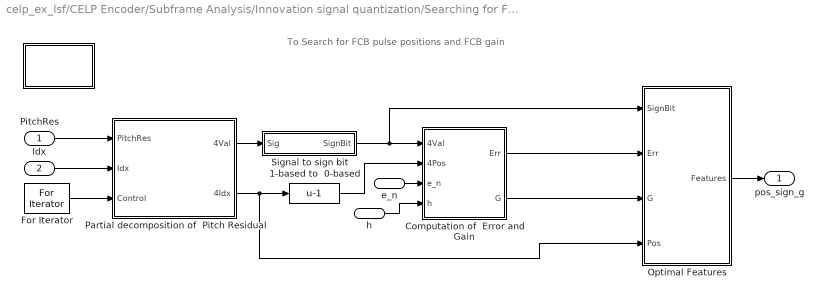
== system celp_ex_lsf/CELP Encoder/Subframe Analysis/Innovation signal quantization/Searching for FCB pulse  positions and FCB gain ==
  note: To Search for FCB pulse positions and FCB gain
  PitchRes : Inport  Port=1  LatchInput=off
  Idx : Inport  Port=2  LatchInput=off
  e_n : Inport  Port=3  LatchInput=off
  h : Inport  Port=4  LatchInput=off
  " " : Subsystem
      mask Type: CELP Coder Demo Info
      mask Display: disp('Info')
  1-based to  0-based : Bias  Bias=-1
  Computation of  Error and Gain : Subsystem
  For Iterator : ForIterator  ResetStates=reset  IterationLimit=37
  Optimal Features : Subsystem
  Partial decomposition of  Pitch Residual : Subsystem
  Signal to sign bit : Subsystem
  pos_sign_g : Outport
  wires:
  1-based to  0-based/1 -> Computation of  Error and Gain/2(4Pos)
  h/1 -> Computation of  Error and Gain/4(h)
  e_n/1 -> Computation of  Error and Gain/3(e_n)
  Signal to sign bit/1(SignBit) -> Computation of  Error and Gain/1(4Val), Optimal Features/1(SignBit)
  Partial decomposition of  Pitch Residual/2(4Idx) -> 1-based to  0-based/1, Optimal Features/4(Pos)
  Partial decomposition of  Pitch Residual/1(4Val) -> Signal to sign bit/1(Sig)
  For Iterator/1 -> Partial decomposition of  Pitch Residual/3(Control)
  Idx/1 -> Partial decomposition of  Pitch Residual/2(Idx)
  PitchRes/1 -> Partial decomposition of  Pitch Residual/1(PitchRes)
  Computation of  Error and Gain/1(Err) -> Optimal Features/2(Err)
  Computation of  Error and Gain/2(G) -> Optimal Features/3(G)
  Optimal Features/1(Features) -> pos_sign_g/1

== system celp_ex_lsf/CELP Encoder/Subframe Analysis/Innovation signal quantization/filter ==
  SigIn2 : Inport  Port=1  LatchInput=off
  K : Inport  Port=2  LatchInput=off
  " " : Subsystem
      mask Type: CELP Coder Demo Info
      mask Display: disp('Info')
  For Iterator : ForIterator  ResetStates=reset  IterationLimit=1  ShowIterationPort=off
  Time-Varying  Synthesis Filter 1/A(z). : dsparch4/Digital Filter  DialogController=dspDDGCreate  DialogControllerArgs=DataTag10  TypePopup=IIR (all poles)  IIRFiltStruct=Direct form II transposed  AllPoleFiltStruct=Lattice AR  FIRFiltStruct=Direct form  CoeffSource=Input port(s)  NumCoeffs=[1 -.95]  DenCoeffs=[1 0.1]  BiQuadCoeffs=[1 0.3 0.4 1 0.1 0.2]  LatticeCoeffs=[0.2 0.4]  denIgnore=off  FiltPerSampPopup=One filter per frame  IC=0  ICnum=0  ICden=0  roundingMode=Floor  overflowMode=off  ScaleValues=1  scaleValueFracLength=14  stageInFracLength=15  stageOutFracLength=15
  SigOut2 : Outport
  wires:
  Time-Varying  Synthesis Filter 1/A(z)./1 -> SigOut2/1
  SigIn2/1 -> Time-Varying  Synthesis Filter 1/A(z)./1
  K/1 -> Time-Varying  Synthesis Filter 1/A(z)./2

== system celp_ex_lsf/CELP Encoder/Subframe Analysis/Pitch Estimation/  ==
  note: Here the following operations occur:
      |
      | 1. The LPC residual signal is obtained by filtering the speech by the
      |     quantized and interpolated LPC analysis filter, A(Z).
      |
      | 2. The parameters specifying the adaptive component of the excitation
      |     (pitch lag and pitch gain) are computed using the open loop pitch estimation
      |     by minimizing the error between the current residual signal and its
      |     scaled-and-delayed version.

== system celp_ex_lsf/CELP Encoder/Subframe Analysis/Pitch Estimation/LPC Residual Calculation ==
  Speech : Inport  Port=1  LatchInput=off
  LSF : Inport  Port=2  LatchInput=off
  LPC to/from RC : dsplp/LPC to//from RC  conversion=LPC to RC  perr=off  stability=off  error=Replace it with 1
  LSF/LSP to LPC Conversion : dsplp/LSF//LSP to LPC Conversion  input=LSF in range (0 pi)
  Time-Varying  Analysis Filter A(z) : dsparch4/Digital Filter  DialogController=dspDDGCreate  DialogControllerArgs=DataTag11  TypePopup=FIR (all zeros)  IIRFiltStruct=Direct form II transposed  AllPoleFiltStruct=Direct form  FIRFiltStruct=Lattice MA  CoeffSource=Input port(s)  NumCoeffs=[1 -.95]  DenCoeffs=[1 0.1]  BiQuadCoeffs=[1 0.3 0.4 1 0.1 0.2]  LatticeCoeffs=[0.2 0.4]  denIgnore=on  FiltPerSampPopup=One filter per frame  IC=0  ICnum=0  ICden=0  roundingMode=Floor  overflowMode=off  ScaleValues=1  scaleValueFracLength=14  stageInFracLength=15  stageOutFracLength=15
  Residual : Outport
  K : Outport  Port=2
  wires:
  LSF/LSP to LPC Conversion/1 -> LPC to/from RC/1
  Speech/1 -> Time-Varying  Analysis Filter A(z)/1
  Time-Varying  Analysis Filter A(z)/1 -> Residual/1
  LSF/1 -> LSF/LSP to LPC Conversion/1
  LPC to/from RC/1 -> Time-Varying  Analysis Filter A(z)/2, K/1

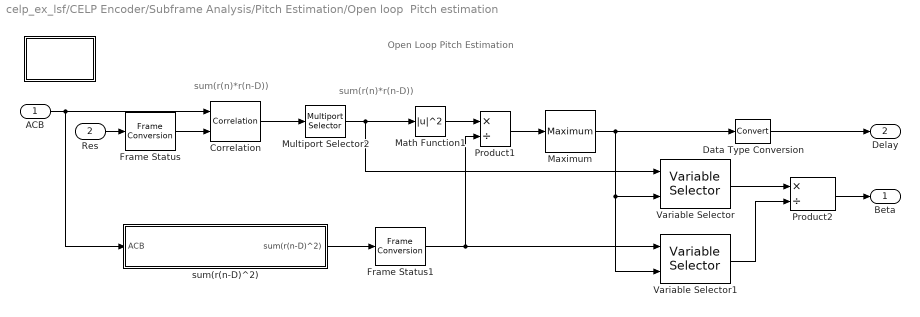
== system celp_ex_lsf/CELP Encoder/Subframe Analysis/Pitch Estimation/Open loop  Pitch estimation ==
  note: sum(r(n)*r(n-D))
  note: sum(r(n)*r(n-D))
  note: Open Loop Pitch Estimation
  ACB : Inport  Port=1  LatchInput=off
  Res : Inport  Port=2  LatchInput=off
  " " : Subsystem
      mask Type: CELP Coder Demo Info
      mask Display: disp('Info')
  Correlation : dspstat3/Correlation  DialogController=dspDDGCreate  DialogControllerArgs=DataTag12  domain=Fastest  roundingMode=Floor  overflowMode=off
  Data Type Conversion : DataTypeConversion  OutDataTypeMode=int32  SaturateOnIntegerOverflow=on  RndMeth=Zero
  Frame Status : FrameConversion  OutFrame=Sample based
  Frame Status1 : FrameConversion  OutFrame=Sample based
  Math Function1 : Math  Operator=magnitude^2  SaturateOnIntegerOverflow=on
  Maximum : dspstat3/Maximum  DialogController=dspDDGCreate  DialogControllerArgs=DataTag13  fcn=Index  reset=None  roundingMode=Floor  overflowMode=off
  Multiport Selector2 : dspindex/Multiport Selector  rowsOrCols=Rows  idxCellArray={40:167}  idxErrMode=Clip Index
  Product1 : Product  Inputs=*/  SaturateOnIntegerOverflow=on
  Product2 : Product  Inputs=*/  SaturateOnIntegerOverflow=on
  Variable Selector : dspindex/Variable Selector  rowsOrCols=Rows  IdxMode=Variable  Elements=[1 3]  ZerOneIdxMode=One-based  errmode=Generate Error
  Variable Selector1 : dspindex/Variable Selector  rowsOrCols=Rows  IdxMode=Variable  Elements=[1 3]  ZerOneIdxMode=One-based  errmode=Generate Error
  sum(r(n-D)^2) : Subsystem  TreatAsAtomicUnit=on
  Beta : Outport
  Delay : Outport  Port=2
  wires:
  Product2/1 -> Beta/1
  Variable Selector/1 -> Product2/1
  Maximum/1 -> Variable Selector1/2, Variable Selector/2, Data Type Conversion/1
  Product1/1 -> Maximum/1
  sum(r(n-D)^2)/1(sum(r(n-D)^2)) -> Frame Status1/1
  Math Function1/1 -> Product1/1
  Res/1 -> Frame Status/1
  ACB/1 -> Correlation/1, sum(r(n-D)^2)/1(ACB)
  Multiport Selector2/1 -> Variable Selector/1, Math Function1/1
  Correlation/1 -> Multiport Selector2/1
  Variable Selector1/1 -> Product2/2
  Frame Status/1 -> Correlation/2
  Frame Status1/1 -> Variable Selector1/1, Product1/2
  Data Type Conversion/1 -> Delay/1

== system celp_ex_lsf/CELP Encoder/Subframe Analysis/Pitch Estimation/Subframe Extraction ==
  Speech : Inport  Port=1  LatchInput=off
  LSF : Inport  Port=2  LatchInput=off
  SubFrIdx : Inport  Orientation=up  Port=3  LatchInput=off
  Frame to subframe : simulink/Math Operations/Reshape  OutputDimensionality=Customize  OutputDimensions=[40,4]
  Variable Selector : dspindex/Variable Selector  rowsOrCols=Columns  IdxMode=Variable  Elements=[1 3]  ZerOneIdxMode=One-based  errmode=Generate Error
  Variable Selector2 : dspindex/Variable Selector  rowsOrCols=Columns  IdxMode=Variable  Elements=[1 3]  ZerOneIdxMode=One-based  errmode=Generate Error
  Speech. : Outport
  LSF. : Outport  Port=2
  wires:
  SubFrIdx/1 -> Variable Selector/2, Variable Selector2/2
  Speech/1 -> Frame to subframe/1
  Variable Selector/1 -> Speech./1
  LSF/1 -> Variable Selector2/1
  Variable Selector2/1 -> LSF./1
  Frame to subframe/1 -> Variable Selector/1

== system celp_ex_lsf/CELP Encoder/Subframe Analysis/Pitch Residual computation/  ==
  note: In this portion of this subsystem, the following operations occur:
      |
      |
      | 1. Pitch gain is quantized using a 6-bit scalar quantizer
      |
      |
      | 2. Pitch delay, the integer-valued pitch lag (values within 1 to 128
      |
      |    inclusive), and the quantized value of pitch gain is used to form the
      |
      |    pitch residual signal. This pitch residual signal is defined as the
      |
      |    difference between the LPC residual signal and its scaled-and-delayed
      |
      |    version.

== system celp_ex_lsf/CELP Encoder/Frame Analysis/LSF Vector Quantization/LSF Split VQ./  ==
  note: In this subsystem, the LPC parameter vectors (LSFs) are quantized using a
      |
      | split vector quantization technique. This technique is a type of product-code
      |
      | vector quantization. In this method, a vector of ten LSFs (LSF1, LSF2, ..., LSF10)
      |
      | is divided into three subvectors. The first subvector contains the first
      |
      | three LSFs (LSF1, LSF2, LSF3). The second subvector contains the next three
      |
      | LSFs (LSF4, LSF5, LSF6). The third subvector contains the remaining four
      |
      | LSFs (LSF7, LSF8, LSF9, LSF10). Each of these subvectors is quantized
      |
      | separately using 10 bits.
      |
      |
      |
      |
      | The three codebooks that correspond to the three subvectors are generated
      |
      | using VQDTool from a training set of 200,000 LSF vectors using the
      |
      | Generalized Lloyd Algorithm (GLA). The weighted mean square error (WMSE)
      |
      | criterion is used as the distortion measure.
      |
      |
      |
      | In this subsystem, the best codebook entry for each subvector is selected
      |
      | based on the minimum weighted Euclidean distance measure. To arrive at the
      |
      | optimal codewords, a sequential search is conducted in each of the three
      |
      | codebooks. All three codewords are concatenated and sorted and thus
      |
      | ordering property in the quantized LSFs is ensured and the stability of the
      |
      | LP filter is guaranteed.

== system celp_ex_lsf/CELP Encoder/Frame Analysis/LSF Vector Quantization/LSF Split VQ./SQ ==
  lspBus : Inport  Port=1  LatchInput=off
  To File : ToFile  Filename=train/lsf.mat  MatrixName=lsf1to10
  wires:
  lspBus/1 -> To File/1

== system celp_ex_lsf/CELP Encoder/Frame Analysis/LSF Vector Quantization/Paliwal Weight  Computation/  ==
  note: Let the unquantized LSF vector is defined as LSF = [LSF1,LSF2, ...,LSF10].
      |
      |
      | The respective weighting vector is W = [w1, w2, ....,w8, 0.8*w9, 0.4*w10].
      |
      |
      | Within this weighting vector, the ith weighting factor, wi, is found using
      |
      | this equation [P(LSFi)]^1.5 (1<=i<=10), where P(f) is the LPC power
      |
      | spectrum associated with the LSF vector as a function of frequency, f].
